simulink model "MRAC_direto"  (Simulink 10.3)
settings: Solver=ode45  StartTime=10  StopTime=20  RelTol=1e-3  AbsTol=1e-6
values from neighbouring files (symbols this model uses):
  As = 0    [simu01.m]    (also in simu02.m = 1; simu03.m; simu04.m = 1; simu05.m)
  DC = 1    [simu01.m]    (also in simu02.m = 2; simu03.m; simu04.m = 2; simu05.m)
  gamma = gamma2    (= 100)    [simu01.m]    (also in simu02.m = gamma2; simu03.m = gamma2; simu04.m = gamma2; simu05.m = gamma2)
  kp = 1    [simu01.m]    (also in simu02.m; simu03.m; simu04.m; simu05.m)
  st = 0.05    [simu01.m]    (also in simu02.m = 0.01; simu03.m = 0.01; simu04.m = 0.01; simu05.m = 0.01)
  theta0 = [0;0]    [simu01.m]    (also in simu02.m; simu03.m; simu04.m; simu05.m)
  ws = 10    [simu01.m]    (also in simu02.m = 5; simu03.m = 5; simu04.m = 5; simu05.m = 5)
libraries: cstblocks x2
settings Model: Creator=Ramon  LastModifiedBy=Lucas  MultithreadedSim=on
settings SolverCC: AutoScaleAbsTol=off
settings DataIOCC: SaveOutput=off  SaveTime=off
settings OptimizationCC: BlockReduction=off  BooleanDataType=off  InitFltsAndDblsToZero=on
settings DebuggingCC: SaveWithParameterizedLinksMsg=none  SignalResolutionControl=TryResolveAllWithWarning  MultiTaskDSMMsg=warning  MultiTaskCondExecSysMsg=none
settings HardwareCC: TargetUnknown=on
settings RTWCC: TemplateMakefile=grt_vc.tmf

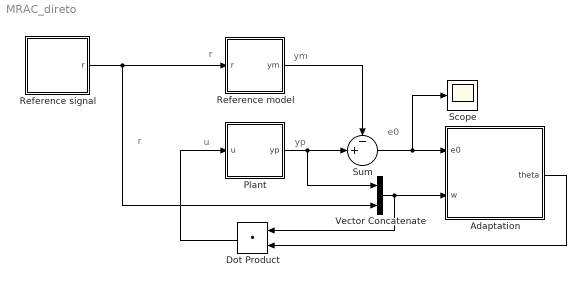
== system MRAC_direto ==
  note: u
  note: r
  note: e0
  note: yp
  note: ym
  note: r
  Adaptation : Subsystem
  Dot Product : DotProduct  InputSameDT=on  OutDataTypeStr=Inherit: Inherit via internal rule
  Plant : Subsystem
  Reference model : Subsystem
  Reference signal : Subsystem
  Scope : Scope
  Sum : Sum  Inputs=-+|  InputSameDT=on  SaturateOnIntegerOverflow=on  OutDataTypeStr=Inherit: Same as first input
  Vector Concatenate : Concatenate
  wires:
  Sum/1 -> Adaptation/1(e0), Scope/1
  Reference model/1(ym) -> Sum/1
  Plant/1(yp) -> Sum/2, Vector Concatenate/1
  Reference signal/1(r) -> Reference model/1(r), Vector Concatenate/2
  Dot Product/1 -> Plant/1(u)
  Adaptation/1(theta) -> Dot Product/2
  Vector Concatenate/1 -> Dot Product/1, Adaptation/2(w)

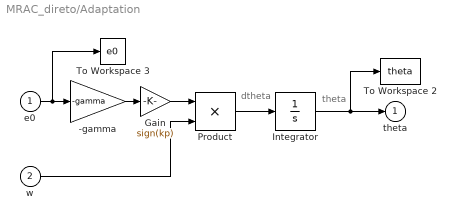
== system MRAC_direto/Adaptation ==
  note: theta
  note: dtheta
  e0 : Inport  PortDimensions=1
  w : Inport  Port=2
  -gamma : Gain  Gain=-gamma  SaturateOnIntegerOverflow=on  OutDataTypeStr=Inherit: Same as input  ParamDataTypeStr=Inherit: Same as input
  Gain : Gain  Gain=sign(kp)
  Integrator : Integrator  InitialCondition=theta0
  Product : Product  InputSameDT=on  RndMeth=Zero  SaturateOnIntegerOverflow=on  OutDataTypeStr=Inherit: Same as first input
  To Workspace 2 : ToWorkspace  VariableName=theta  SampleTime=st
  To Workspace 3 : ToWorkspace  VariableName=e0  SampleTime=st
  theta : Outport  InitialOutput=0  VectorParamsAs1DForOutWhenUnconnected=off
  wires:
  Integrator/1 -> To Workspace 2/1, theta/1
  Gain/1 -> Product/1
  w/1 -> Product/2
  e0/1 -> -gamma/1, To Workspace 3/1
  Product/1 -> Integrator/1
  -gamma/1 -> Gain/1

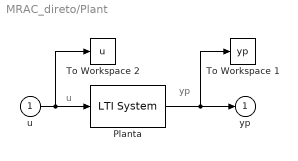
== system MRAC_direto/Plant ==
  note: yp
  note: u
  u : Inport
  Planta : cstblocks/LTI System  sys=P  IC=x0
  To Workspace 1 : ToWorkspace  VariableName=yp  SampleTime=st
  To Workspace 2 : ToWorkspace  VariableName=u  SampleTime=st
  yp : Outport  InitialOutput=0  VectorParamsAs1DForOutWhenUnconnected=off
  wires:
  u/1 -> To Workspace 2/1, Planta/1
  Planta/1 -> yp/1, To Workspace 1/1

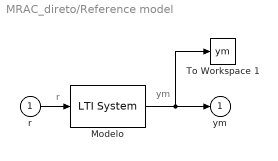
== system MRAC_direto/Reference model ==
  note: r
  note: ym
  r : Inport
  Modelo : cstblocks/LTI System  sys=M  IC=xm0
  To Workspace 1 : ToWorkspace  VariableName=ym  SampleTime=st
  ym : Outport  InitialOutput=0  VectorParamsAs1DForOutWhenUnconnected=off
  wires:
  Modelo/1 -> To Workspace 1/1, ym/1
  r/1 -> Modelo/1

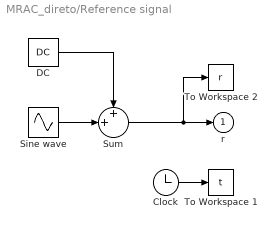
== system MRAC_direto/Reference signal ==
  Clock : Clock
  DC : Constant  Value=DC
  Sine wave : Sin  Amplitude=As  Frequency=ws  SampleTime=0
  Sum : Sum  Inputs=++|  InputSameDT=on  SaturateOnIntegerOverflow=on  OutDataTypeStr=Inherit: Same as first input
  To Workspace 1 : ToWorkspace  VariableName=t  SampleTime=st
  To Workspace 2 : ToWorkspace  VariableName=r  SampleTime=st
  r : Outport  InitialOutput=0  VectorParamsAs1DForOutWhenUnconnected=off
  wires:
  DC/1 -> Sum/1
  Sum/1 -> r/1, To Workspace 2/1
  Clock/1 -> To Workspace 1/1
  Sine wave/1 -> Sum/2
